simulink model "LAB1"  (R2024a)
settings: Solver=FixedStepDiscrete  StartTime=0.0  StopTime=100  RelTol=1e-3
settings Model: Creator=VICTUS  LastModifiedBy=VICTUS

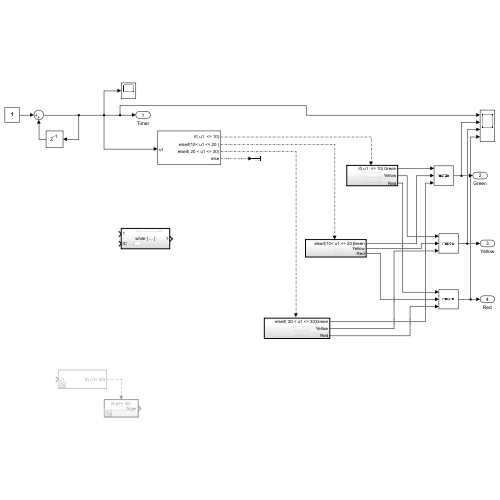
[thumbnail: Simulink's stored preview of the top-level diagram]
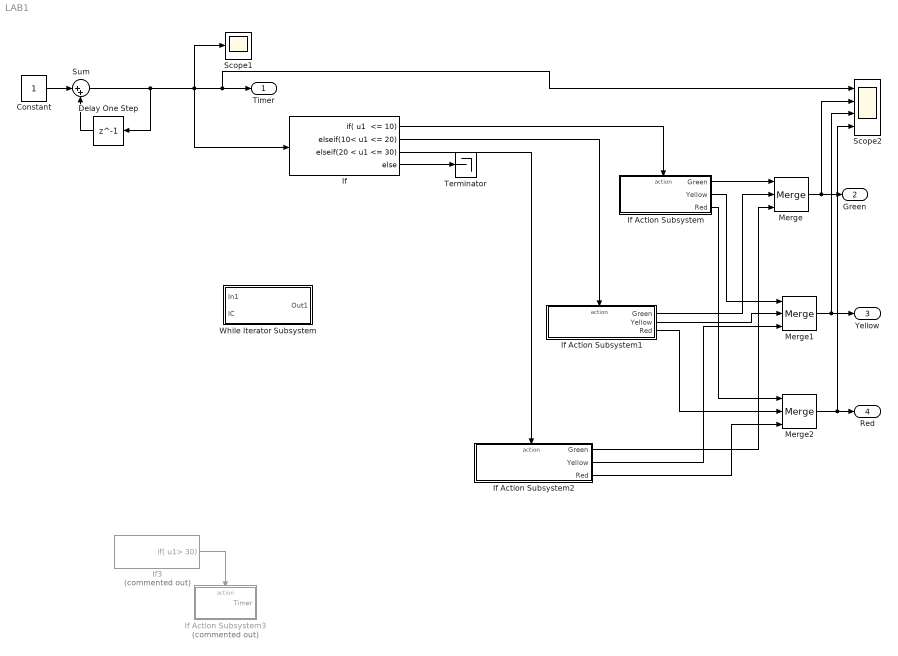
== system LAB1 ==
  Constant : Constant
  Delay One Step : Delay  DelayLength=1
  If : If  IfExpression="u1  <= 10"  ElseIfExpressions=10< u1 <= 20 , 20 < u1 <= 30
  If Action Subsystem : Subsystem  TreatAsAtomicUnit=on
  If Action Subsystem1 : Subsystem  TreatAsAtomicUnit=on
  If Action Subsystem2 : Subsystem  TreatAsAtomicUnit=on
  If Action Subsystem3 : Subsystem  Commented=on  TreatAsAtomicUnit=on
  If3 : If  Commented=on  IfExpression=u1> 30  ShowElse=off
  Merge : Merge  Inputs=3
  Merge1 : Merge  Inputs=3
  Merge2 : Merge  Inputs=3
  Scope1 : Scope
  Scope2 : Scope  NumInputPorts=4
  Sum : Sum  Inputs=|++
  Terminator : Terminator
  While Iterator Subsystem : Subsystem  TreatAsAtomicUnit=on
  Timer : Outport  InitialOutput=[0]
  Green : Outport  Port=2
  Yellow : Outport  Port=3
  Red : Outport  Port=4
  wires:
  If/1 -> If Action Subsystem/Action
  If/3 -> If Action Subsystem2/Action
  If3/1 -> If Action Subsystem3/Action
  Constant/1 -> Sum/1
  Sum/1 -> If/1, Scope1/1, Scope2/1, Timer/1, Delay One Step/1
  Delay One Step/1 -> Sum/2
  If/2 -> If Action Subsystem1/Action
  Merge/1 -> Scope2/2, Green/1
  If Action Subsystem/1(Green) -> Merge/1
  If Action Subsystem1/1(Green) -> Merge/2
  If Action Subsystem2/1(Green) -> Merge/3
  Merge1/1 -> Scope2/3, Yellow/1
  If Action Subsystem/2(Yellow) -> Merge1/1
  If Action Subsystem1/2(Yellow) -> Merge1/2
  If Action Subsystem2/2(Yellow) -> Merge1/3
  Merge2/1 -> Scope2/4, Red/1
  If Action Subsystem/3(Red) -> Merge2/1
  If Action Subsystem1/3(Red) -> Merge2/2
  If Action Subsystem2/3(Red) -> Merge2/3
  If/4 -> Terminator/1

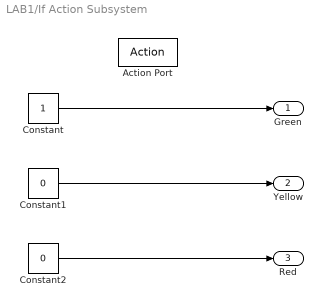
== system LAB1/If Action Subsystem ==
  Action Port : ActionPort  ActionPortLabel="if( u1  <= 10)"
  Constant : Constant
  Constant1 : Constant  Value=0
  Constant2 : Constant  Value=0
  Green : Outport  InitialOutput=0
  Yellow : Outport  Port=2
  Red : Outport  Port=3
  wires:
  Constant/1 -> Green/1
  Constant1/1 -> Yellow/1
  Constant2/1 -> Red/1

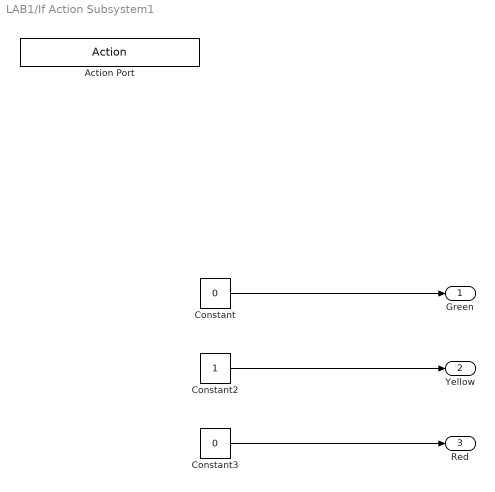
== system LAB1/If Action Subsystem1 ==
  Action Port : ActionPort  ActionPortLabel=elseif(10< u1 <= 20 )
  Constant : Constant  Value=0
  Constant2 : Constant
  Constant3 : Constant  Value=0
  Green : Outport  InitialOutput=0
  Yellow : Outport  Port=2
  Red : Outport  Port=3
  wires:
  Constant3/1 -> Red/1
  Constant2/1 -> Yellow/1
  Constant/1 -> Green/1

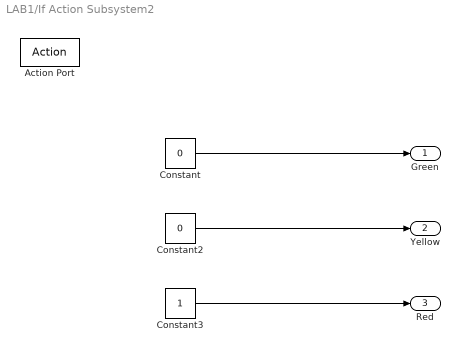
== system LAB1/If Action Subsystem2 ==
  Action Port : ActionPort  ActionPortLabel=elseif( 20 < u1 <= 30)
  Constant : Constant  Value=0
  Constant2 : Constant  Value=0
  Constant3 : Constant
  Green : Outport  InitialOutput=0
  Yellow : Outport  Port=2
  Red : Outport  Port=3
  wires:
  Constant/1 -> Green/1
  Constant2/1 -> Yellow/1
  Constant3/1 -> Red/1

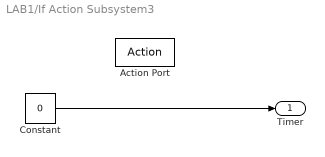
== system LAB1/If Action Subsystem3 ==
  Action Port : ActionPort  ActionPortLabel=if( u1> 30)
  Constant : Constant  Value=0
  Timer : Outport
  wires:
  Constant/1 -> Timer/1

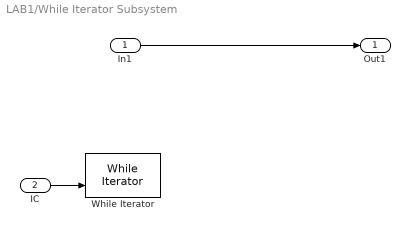
== system LAB1/While Iterator Subsystem ==
  In1 : Inport
  IC : Inport  Port=2
  While Iterator : WhileIterator
  Out1 : Outport
  wires:
  IC/1 -> While Iterator/2
  In1/1 -> Out1/1
